simulink model "carModelVConst"  (R2020b)
settings: Solver=VariableStepAuto  StartTime=0.0  StopTime=10.0  RelTol=1e-3
undefined symbols (not defined in the file or in its folder): carDyanamics, magnitude
settings Model: Creator=Yuto  LastModifiedBy=Yuto

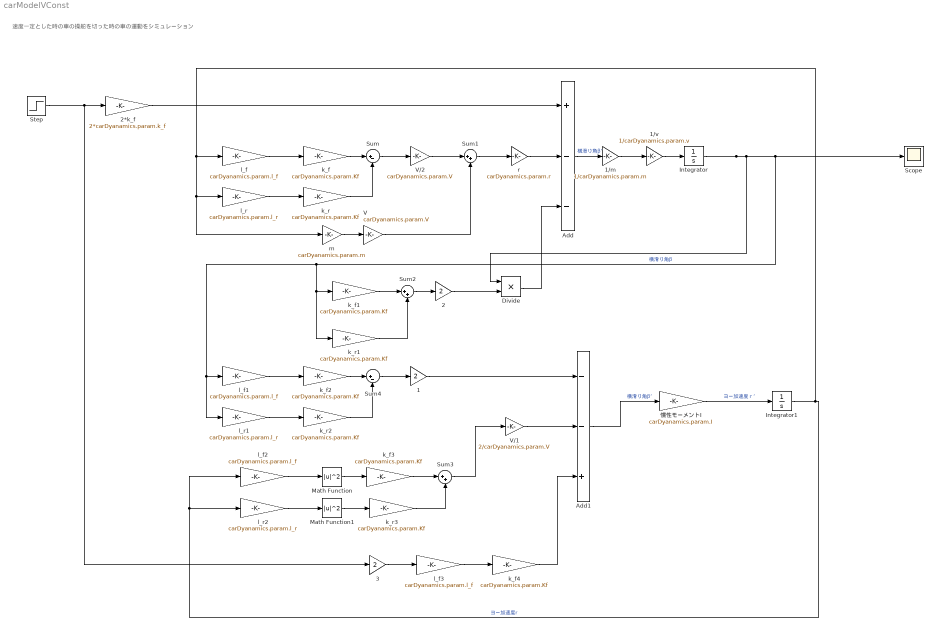
== system carModelVConst ==
  note: 速度一定とした時の車の操舵を切った時の車の運動をシミュレーション
  1 : Gain  Gain=2
  1/m : Gain  Gain=1/carDyanamics.param.m
  1/v : Gain  Gain=1/carDyanamics.param.v
  2 : Gain  Gain=2
  2*k_f : Gain  Gain=2*carDyanamics.param.k_f
  3 : Gain  Gain=2
  Add : Sum  Inputs=+--
  Add1 : Sum  Inputs=--+
  Divide : Product  Inputs=**
  Integrator : Integrator
  Integrator1 : Integrator
  Math Function : Math  Operator=magnitude^2  SaturateOnIntegerOverflow=on
  Math Function1 : Math  Operator=magnitude^2  SaturateOnIntegerOverflow=on
  Scope : Scope
  Step : Step  SampleTime=0
  Sum : Sum  Inputs=|+-
  Sum1 : Sum  Inputs=|++
  Sum2 : Sum  Inputs=|++
  Sum3 : Sum  Inputs=|++
  Sum4 : Sum  Inputs=|+-
  V : Gain  Gain=carDyanamics.param.V
  V/1 : Gain  Gain=2/carDyanamics.param.V
  V/2 : Gain  Gain=carDyanamics.param.V
  k_f{,1..4} (5 alike) : Gain  Gain=carDyanamics.param.Kf
  k_r{,1..3} (4 alike) : Gain  Gain=carDyanamics.param.Kf
  l_f{,1..3} (4 alike) : Gain  Gain=carDyanamics.param.l_f
  l_r : Gain  Gain=carDyanamics.param.l_r
  l_r1 : Gain  Gain=carDyanamics.param.l_r
  l_r2 : Gain  Gain=carDyanamics.param.l_r
  m : Gain  Gain=carDyanamics.param.m
  r : Gain  Gain=carDyanamics.param.r
  慣性モーメントI : Gain  Gain=carDyanamics.param.I
  wires:
  Integrator/1 -> Divide/1, k_r1/1, k_f1/1, l_r1/1, l_f1/1, Scope/1  "横滑り角β"
  m/1 -> V/1
  V/1 -> Sum1/2
  l_f/1 -> k_f/1
  k_f/1 -> Sum/1
  k_r/1 -> Sum/2
  l_r/1 -> k_r/1
  Sum/1 -> V/2/1
  V/2/1 -> Sum1/1
  k_f1/1 -> Sum2/1
  k_r1/1 -> Sum2/2
  Sum2/1 -> 2/1
  1/m/1 -> 1/v/1
  Sum1/1 -> r/1
  r/1 -> Add/2
  2/1 -> Divide/2
  Divide/1 -> Add/3
  Step/1 -> 3/1, 2*k_f/1
  慣性モーメントI/1 -> Integrator1/1  "ヨー加速度ｒ’"
  Integrator1/1 -> l_r2/1, l_f2/1, l_f/1, m/1, l_r/1  "ヨー加速度r"
  Sum4/1 -> 1/1
  k_r2/1 -> Sum4/2
  k_f2/1 -> Sum4/1
  l_f1/1 -> k_f2/1
  l_r1/1 -> k_r2/1
  2*k_f/1 -> Add/1
  1/1 -> Add1/1
  l_f2/1 -> Math Function/1
  Math Function/1 -> k_f3/1
  l_r2/1 -> Math Function1/1
  Math Function1/1 -> k_r3/1
  k_f3/1 -> Sum3/1
  k_r3/1 -> Sum3/2
  Sum3/1 -> V/1/1
  V/1/1 -> Add1/2
  Add1/1 -> 慣性モーメントI/1  "横滑り角β’"
  Add/1 -> 1/m/1  "横滑り角β’"
  1/v/1 -> Integrator/1
  l_f3/1 -> k_f4/1
  k_f4/1 -> Add1/3
  3/1 -> l_f3/1
